simulink model "simeso"  (R2022b)
settings: Solver=FixedStepAuto  StartTime=0.0  StopTime=1  FixedStep=1/10000  RelTol=1e-3
settings Model: Creator=zzy  LastModifiedBy=zzy

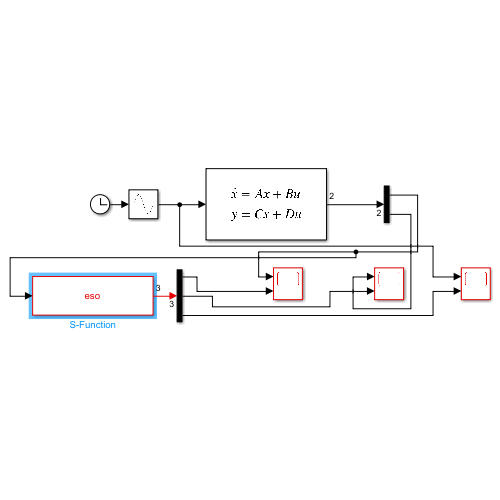
[thumbnail: Simulink's stored preview of the top-level diagram]
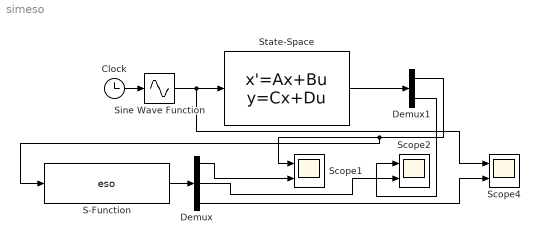
== system simeso ==
  Clock : Clock
  Demux : Demux  Outputs=3
  Demux1 : Demux  Outputs=2
  S-Function : S-Function  FunctionName=eso  SFunctionDeploymentMode=off  EnableBusSupport=off
  Scope1 : Scope  NumInputPorts=2
  Scope2 : Scope  NumInputPorts=2
  Scope4 : Scope  NumInputPorts=2
  Sine Wave Function : Sin  TimeSource=Use external signal  Frequency=100  SampleTime=0
  State-Space : StateSpace  A=[0 1;0 0]  B=[0;1]  C=[1 0 ; 0 1]  D="[0  ; 0]"  InitialCondition=0
  wires:
  Demux1/1 -> S-Function/1, Scope1/1
  Sine Wave Function/1 -> Scope4/1, State-Space/1
  Clock/1 -> Sine Wave Function/1
  S-Function/1 -> Demux/1
  Demux/3 -> Scope4/2
  State-Space/1 -> Demux1/1
  Demux/1 -> Scope1/2
  Demux1/2 -> Scope2/1
  Demux/2 -> Scope2/2
